simulink model "MySimplifiedTestingModel_20x2810x29"  (R2023a)
settings: Solver=ode1  StartTime=0.0  StopTime=inf  FixedStep=0.001  RelTol=1e-3
PostLoadFcn:
  | , if any(exist('dsrtsu_mdlpostloadfcn', 'file') ~= 0), dsrtsu_mdlpostloadfcn('Execute', bdroot); end,
InitFcn:
  | , if any(exist('rtifpga_mdlclblib', 'file') ~= 0), rtifpga_mdlclblib('Init', bdroot); end,
undefined symbols (not defined in the file or in its folder): START, STOP
libraries: rti1202serlib x11, simulink x6
(part 2 of 3)

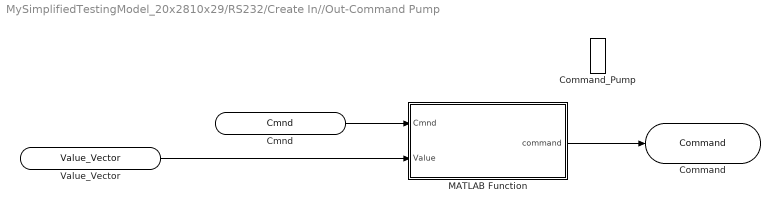
== system MySimplifiedTestingModel_20x2810x29/RS232/Create In//Out-Command Pump ==
  Command_Pump : TriggerPort  TriggerType=function-call  IsSimulinkFunction=on  FunctionName=Command_Pump  VariantControl=(inherit)
  MATLAB Function : MATLAB Function  TreatAsAtomicUnit=on
  Cmnd : ArgIn  ArgumentName=Cmnd
  Value_Vector : ArgIn  Port=2  ArgumentName=Value_Vector
  Command : ArgOut  OutDataTypeStr=uint8  PortDimensions=[1,13]  ArgumentName=Command
  wires:
  Value_Vector/1 -> MATLAB Function/2(Value)
  Cmnd/1 -> MATLAB Function/1(Cmnd)
  MATLAB Function/1(command) -> Command/1

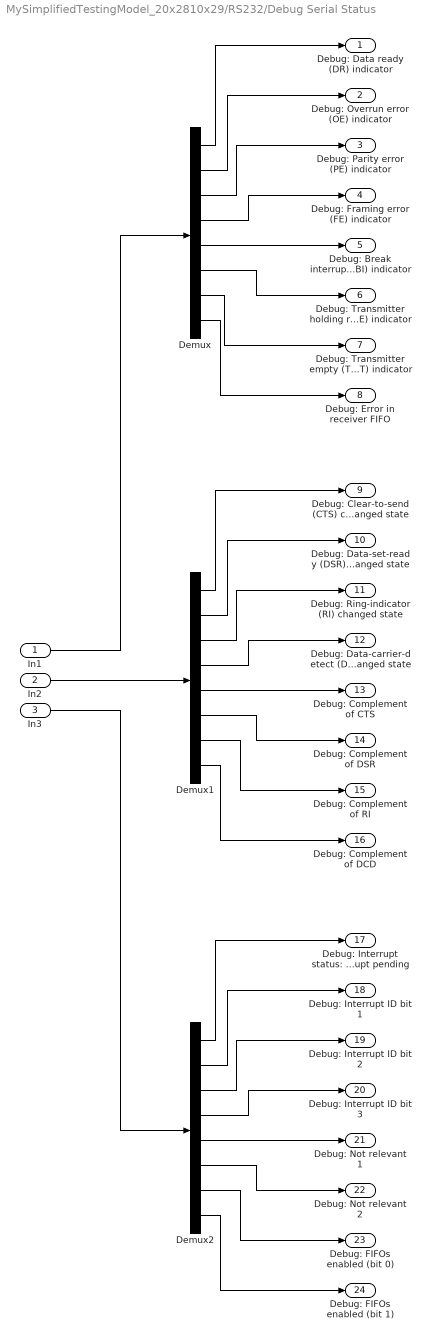
== system MySimplifiedTestingModel_20x2810x29/RS232/Debug Serial Status ==
  In1 : Inport
  In2 : Inport  Port=2
  In3 : Inport  Port=3
  Demux : Demux  Outputs=8
  Demux1 : Demux  Outputs=8
  Demux2 : Demux  Outputs=8
  Debug: Data ready (DR) indicator : Outport
  Debug: Overrun error (OE) indicator : Outport  Port=2
  Debug: Parity error (PE) indicator : Outport  Port=3
  Debug: Framing error (FE) indicator : Outport  Port=4
  Debug: Break interrupt (BI) indicator : Outport  Port=5
  Debug: Transmitter holding register empty (THRE) indicator : Outport  Port=6
  Debug: Transmitter empty (TEMT) indicator : Outport  Port=7
  Debug: Error in receiver FIFO : Outport  Port=8
  Debug: Clear-to-send (CTS) changed state : Outport  Port=9
  Debug: Data-set-ready (DSR) changed state : Outport  Port=10
  Debug: Ring-indicator (RI) changed state : Outport  Port=11
  Debug: Data-carrier-detect (DCD) changed state : Outport  Port=12
  Debug: Complement of CTS : Outport  Port=13
  Debug: Complement of DSR : Outport  Port=14
  Debug: Complement of RI : Outport  Port=15
  Debug: Complement of DCD : Outport  Port=16
  Debug: Interrupt status: 0 if interrupt pending : Outport  Port=17
  Debug: Interrupt ID bit 1 : Outport  Port=18
  Debug: Interrupt ID bit 2 : Outport  Port=19
  Debug: Interrupt ID bit 3 : Outport  Port=20
  Debug: Not relevant 1 : Outport  Port=21
  Debug: Not relevant 2 : Outport  Port=22
  Debug: FIFOs enabled (bit 0) : Outport  Port=23
  Debug: FIFOs enabled (bit 1) : Outport  Port=24
  wires:
  Demux/3 -> Debug: Parity error (PE) indicator/1
  Demux2/4 -> Debug: Interrupt ID bit 3/1
  Demux1/8 -> Debug: Complement of DCD/1
  Demux2/5 -> Debug: Not relevant 1/1
  Demux2/2 -> Debug: Interrupt ID bit 1/1
  Demux/1 -> Debug: Data ready (DR) indicator/1
  In2/1 -> Demux1/1
  Demux1/2 -> Debug: Data-set-ready (DSR) changed state/1
  In1/1 -> Demux/1
  Demux2/7 -> Debug: FIFOs enabled (bit 0)/1
  Demux2/1 -> Debug: Interrupt status: 0 if interrupt pending/1
  Demux2/6 -> Debug: Not relevant 2/1
  Demux2/3 -> Debug: Interrupt ID bit 2/1
  Demux1/7 -> Debug: Complement of RI/1
  Demux1/1 -> Debug: Clear-to-send (CTS) changed state/1
  Demux1/6 -> Debug: Complement of DSR/1
  Demux1/4 -> Debug: Data-carrier-detect (DCD) changed state/1
  Demux1/5 -> Debug: Complement of CTS/1
  Demux1/3 -> Debug: Ring-indicator (RI) changed state/1
  Demux/2 -> Debug: Overrun error (OE) indicator/1
  Demux2/8 -> Debug: FIFOs enabled (bit 1)/1
  Demux/6 -> Debug: Transmitter holding register empty (THRE) indicator/1
  Demux/5 -> Debug: Break interrupt (BI) indicator/1
  Demux/4 -> Debug: Framing error (FE) indicator/1
  Demux/8 -> Debug: Error in receiver FIFO/1
  Demux/7 -> Debug: Transmitter empty (TEMT) indicator/1
  In3/1 -> Demux2/1

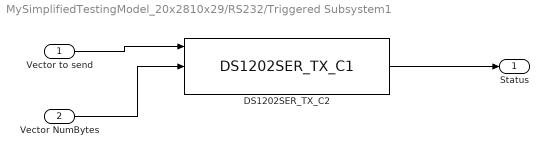
== system MySimplifiedTestingModel_20x2810x29/RS232/Triggered Subsystem1 ==
  Vector to send : Inport
  Vector NumBytes : Inport  Port=2
  DS1202SER_TX_C2 : rti1202serlib/DS1202SER_TX_C1  Reserved1=[]  Reserved2=[]  Reserved3=[]  Reserved4=[]  DSProperties=struct('RTI',struct('IOBoardType',{{'DS1202','SER'}},'SlaveProcessor','NONE','Version',uint32(1),'BlockType',struct('isSLSource',uint8(1),'isSLSink',uint8(1),'isHWSource',uint8(1),'isHWSink',uint8(0),'isSetup',uint8(0),'isInline',uint8(1),'isNonInline',uint8(0),'isInterrupt',uint8(0),'isChannelwise',uint8(1)),'UnitType','GENSER','Identifier','TRANSMIT','DialogType','ML','BlockSet','NONE'))  RTIBlockInterface=struct('BlockName',struct('Token',{{'DS1202SER_TX_C'}},'BlockParam',{{'ChannelNo'}}),'InputPortsWidth',int32([13 1]),'InputPortsActive',[1 1],'InputPortsDataType',{{'SS_UINT8','SS_UINT32'}},'InputPortsName',{{'TXBytes','NumBytes'}},'OutputPortsWidth',int32([1 1]),'OutputPortsActive',[0 1],'OutputPortsDataType',{{'SS_UINT32','SS_INT32'}},'OutputPortsName',{{'NumTXBytes','Status'}},'BlockDisplay',{{['Serial Transmit'],'center'}},'IconTransparency','on','ParameterTunableNames',{{'BytesRefNumOf'}},'InitLevel',2,'DialogFcn','guigensertransmit','MaskDescription',['To write data to the UART SW FIFO.'])  RTIBlockParameters=struct('BoardNo',{{1,'ON',[1 1]}},'ChannelNo',{{2,'ON',[1 2]}},'ChannelNumOf',{{2,'OFF',[]}},'TransmitFifoOverrunMode',{{1,'OFF',[]}},'ParamTunableMode',{{1,'OFF',[]}},'BytesRefNumOfT',{{'1','OFF',[1 inf]}},'BytesRefNumOfNT',{{'1','OFF',[1 inf]}},'BytesRefNumOfMax',{{'13','OFF',[1 inf]}},'BytesRefNumOfMode',{{0,'OFF',[]}},'BytesActNumOfMode',{{0,'OFF',[]}},'TransmissionStatusMode',{{1,'OFF',[]}},'FifoSizeDefault',{{64,'OFF',[]}},'TLCFileName',{{'rtigensertransmit','OFF',[]}})  RTISFcnParameters=struct('BoardNo','double','ChannelNo','double','ChannelNumOf','double','TransmitFifoOverrunMode','double','ParamTunableMode','double','BytesRefNumOfT','double','BytesRefNumOfNT','double','BytesRefNumOfMax','double','BytesRefNumOfMode','double','BytesActNumOfMode','double','TransmissionStatusMode','double','TLCFileName','char')  RTIBlockParaDefault=struct('BoardNo',1,'ChannelNo',1,'ChannelNumOf',2,'TransmitFifoOverrunMode',1,'ParamTunableMode',1,'BytesRefNumOfT',1,'BytesRefNumOfNT',1,'BytesRefNumOfMax',1,'BytesRefNumOfMode',0,'BytesActNumOfMode',1,'TransmissionStatusMode',1,'FifoSizeDefault',64,'TLCFileName','rtigensertransmit')
  Status : Outport
  wires:
  DS1202SER_TX_C2/1 -> Status/1
  Vector NumBytes/1 -> DS1202SER_TX_C2/2
  Vector to send/1 -> DS1202SER_TX_C2/1

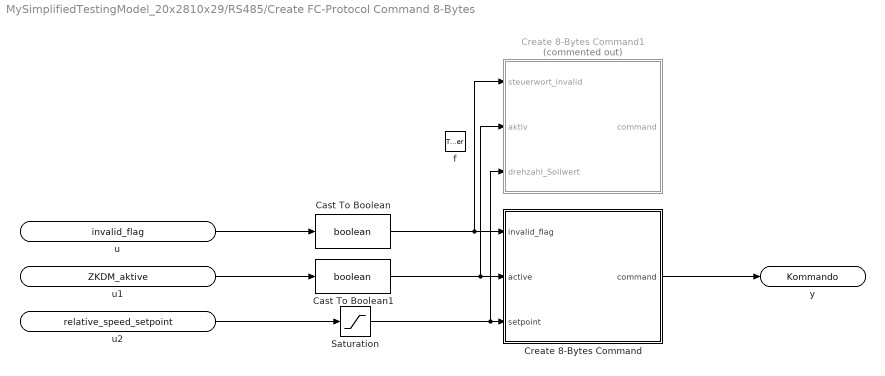
== system MySimplifiedTestingModel_20x2810x29/RS485/Create FC-Protocol Command 8-Bytes ==
  f : TriggerPort  TriggerType=function-call  IsSimulinkFunction=on  FunctionName=FC_Command_8Bytes  VariantControl=(inherit)
  Cast To Boolean : DataTypeConversion  OutDataTypeStr=boolean  SaturateOnIntegerOverflow=off  RndMeth=Floor
  Cast To Boolean1 : DataTypeConversion  OutDataTypeStr=boolean  SaturateOnIntegerOverflow=off  RndMeth=Floor
  Create 8-Bytes Command : MATLAB Function  TreatAsAtomicUnit=on
  Create 8-Bytes Command1 : MATLAB Function  Commented=on  TreatAsAtomicUnit=on
  Saturation : Saturate  UpperLimit=100  LowerLimit=0
  u : ArgIn  DisableCoverage=on  ArgumentName=invalid_flag
  u1 : ArgIn  DisableCoverage=on  Port=2  ArgumentName=ZKDM_aktive
  u2 : ArgIn  DisableCoverage=on  Port=3  ArgumentName=relative_speed_setpoint
  y : ArgOut  DisableCoverage=on  OutDataTypeStr=uint8  PortDimensions=[1, 63]  ArgumentName=Kommando
  wires:
  Saturation/1 -> Create 8-Bytes Command/3(setpoint), Create 8-Bytes Command1/3(drehzahl_Sollwert)
  Cast To Boolean1/1 -> Create 8-Bytes Command/2(active), Create 8-Bytes Command1/2(aktiv)
  Cast To Boolean/1 -> Create 8-Bytes Command/1(invalid_flag), Create 8-Bytes Command1/1(steuerwort_invalid)
  u2/1 -> Saturation/1
  u1/1 -> Cast To Boolean1/1
  u/1 -> Cast To Boolean/1
  Create 8-Bytes Command/1(command) -> y/1

== system MySimplifiedTestingModel_20x2810x29/RS485/Konfiguration für kommunikation ZKDM ==
  Trigger : TriggerPort  VariantControl=(inherit)
  System Outputs : Subsystem  mask(System Outputs){ShowInLibBrowser=0}
      mask prompts: ShowInLibBrowser "Simulink:masks:CustCodeMaskParam1_MP"
      settings: CopyFcn=cccopyfcn(gcb)  OpenFcn=ccopenfcn('System Outputs Function')
      mask Help: eval('feval(''rtwprivate'',''rtwhelpview'',''rtw_sys_outputs_block'')');
      mask DialogControl ShowInLibBrowser Prompt: Mask Parameter 1:
      mask Display: disp('System\nOutputs');

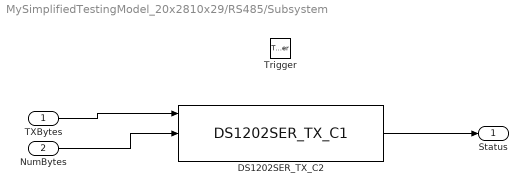
== system MySimplifiedTestingModel_20x2810x29/RS485/Subsystem ==
  TXBytes : Inport
  NumBytes : Inport  Port=2
  Trigger : TriggerPort  VariantControl=(inherit)  PortDimensions=1
  DS1202SER_TX_C2 : rti1202serlib/DS1202SER_TX_C1  Reserved1=[]  Reserved2=[]  Reserved3=[]  Reserved4=[]  DSProperties=struct('RTI',struct('IOBoardType',{{'DS1202','SER'}},'SlaveProcessor','NONE','Version',uint32(1),'BlockType',struct('isSLSource',uint8(1),'isSLSink',uint8(1),'isHWSource',uint8(1),'isHWSink',uint8(0),'isSetup',uint8(0),'isInline',uint8(1),'isNonInline',uint8(0),'isInterrupt',uint8(0),'isChannelwise',uint8(1)),'UnitType','GENSER','Identifier','TRANSMIT','DialogType','ML','BlockSet','NONE'))  RTIBlockInterface=struct('BlockName',struct('Token',{{'DS1202SER_TX_C'}},'BlockParam',{{'ChannelNo'}}),'InputPortsWidth',int32([63 1]),'InputPortsActive',[1 1],'InputPortsDataType',{{'SS_UINT8','SS_UINT32'}},'InputPortsName',{{'TXBytes','NumBytes'}},'OutputPortsWidth',int32([1 1]),'OutputPortsActive',[0 1],'OutputPortsDataType',{{'SS_UINT32','SS_INT32'}},'OutputPortsName',{{'NumTXBytes','Status'}},'BlockDisplay',{{['Serial Transmit'],'center'}},'IconTransparency','on','ParameterTunableNames',{{'BytesRefNumOf'}},'InitLevel',2,'DialogFcn','guigensertransmit','MaskDescription',['To write data to the UART SW FIFO.'])  RTIBlockParameters=struct('BoardNo',{{1,'ON',[1 1]}},'ChannelNo',{{2,'ON',[1 2]}},'ChannelNumOf',{{2,'OFF',[]}},'TransmitFifoOverrunMode',{{1,'OFF',[]}},'ParamTunableMode',{{1,'OFF',[]}},'BytesRefNumOfT',{{'1','OFF',[1 inf]}},'BytesRefNumOfNT',{{'1','OFF',[1 inf]}},'BytesRefNumOfMax',{{'63','OFF',[1 inf]}},'BytesRefNumOfMode',{{0,'OFF',[]}},'BytesActNumOfMode',{{0,'OFF',[]}},'TransmissionStatusMode',{{1,'OFF',[]}},'FifoSizeDefault',{{64,'OFF',[]}},'TLCFileName',{{'rtigensertransmit','OFF',[]}})  RTISFcnParameters=struct('BoardNo','double','ChannelNo','double','ChannelNumOf','double','TransmitFifoOverrunMode','double','ParamTunableMode','double','BytesRefNumOfT','double','BytesRefNumOfNT','double','BytesRefNumOfMax','double','BytesRefNumOfMode','double','BytesActNumOfMode','double','TransmissionStatusMode','double','TLCFileName','char')  RTIBlockParaDefault=struct('BoardNo',1,'ChannelNo',1,'ChannelNumOf',2,'TransmitFifoOverrunMode',1,'ParamTunableMode',1,'BytesRefNumOfT',1,'BytesRefNumOfNT',1,'BytesRefNumOfMax',1,'BytesRefNumOfMode',0,'BytesActNumOfMode',1,'TransmissionStatusMode',1,'FifoSizeDefault',64,'TLCFileName','rtigensertransmit')
  Status : Outport
  wires:
  TXBytes/1 -> DS1202SER_TX_C2/1
  DS1202SER_TX_C2/1 -> Status/1
  NumBytes/1 -> DS1202SER_TX_C2/2

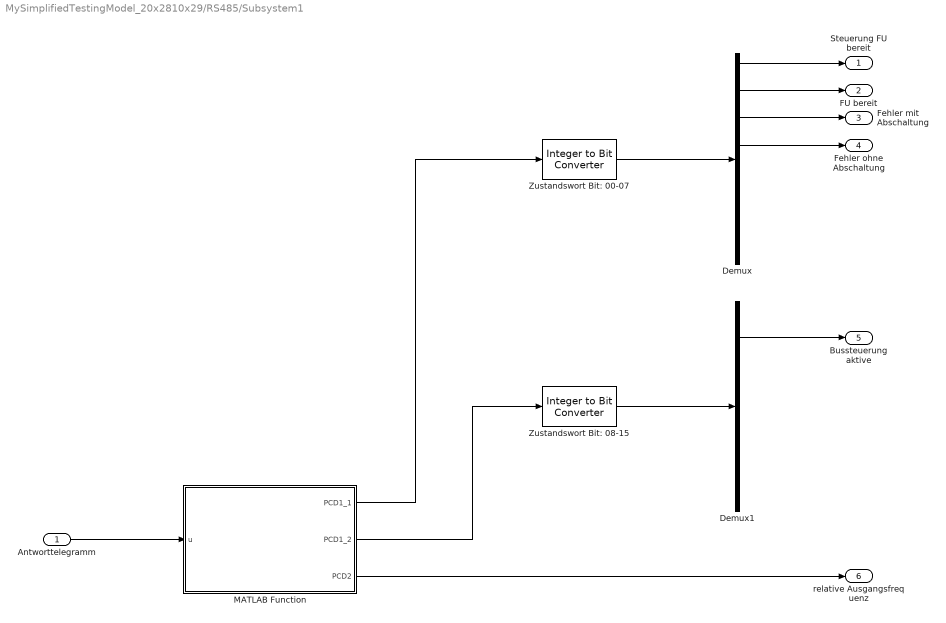
== system MySimplifiedTestingModel_20x2810x29/RS485/Subsystem1 ==
  Antworttelegramm : Inport
  Demux : Demux  Outputs=8
  Demux1 : Demux  Outputs=8
  MATLAB Function : MATLAB Function  TreatAsAtomicUnit=on
  Zustandswort Bit: 00-07 : simulink/Logic and Bit Operations/Integer to Bit Converter  nbits=8  signedInputValues=Unsigned  bitOrder=MSB first  outDtype=boolean
  Zustandswort Bit: 08-15 : simulink/Logic and Bit Operations/Integer to Bit Converter  nbits=8  signedInputValues=Unsigned  bitOrder=MSB first  outDtype=boolean
  Steuerung FU bereit : Outport
  FU bereit : Outport  Port=2
  Fehler mit Abschaltung : Outport  Port=3
  Fehler ohne Abschaltung : Outport  Port=4
  Bussteuerung aktive : Outport  Port=5
  relative Ausgangsfrequenz : Outport  Port=6
  wires:
  MATLAB Function/3(PCD2) -> relative Ausgangsfrequenz/1
  MATLAB Function/2(PCD1_2) -> Zustandswort Bit: 08-15/1
  MATLAB Function/1(PCD1_1) -> Zustandswort Bit: 00-07/1
  Demux1/2 -> Bussteuerung aktive/1
  Zustandswort Bit: 08-15/1 -> Demux1/1
  Zustandswort Bit: 00-07/1 -> Demux/1
  Demux/4 -> Fehler ohne Abschaltung/1
  Demux/3 -> Fehler mit Abschaltung/1
  Demux/2 -> FU bereit/1
  Demux/1 -> Steuerung FU bereit/1
  Antworttelegramm/1 -> MATLAB Function/1(u)

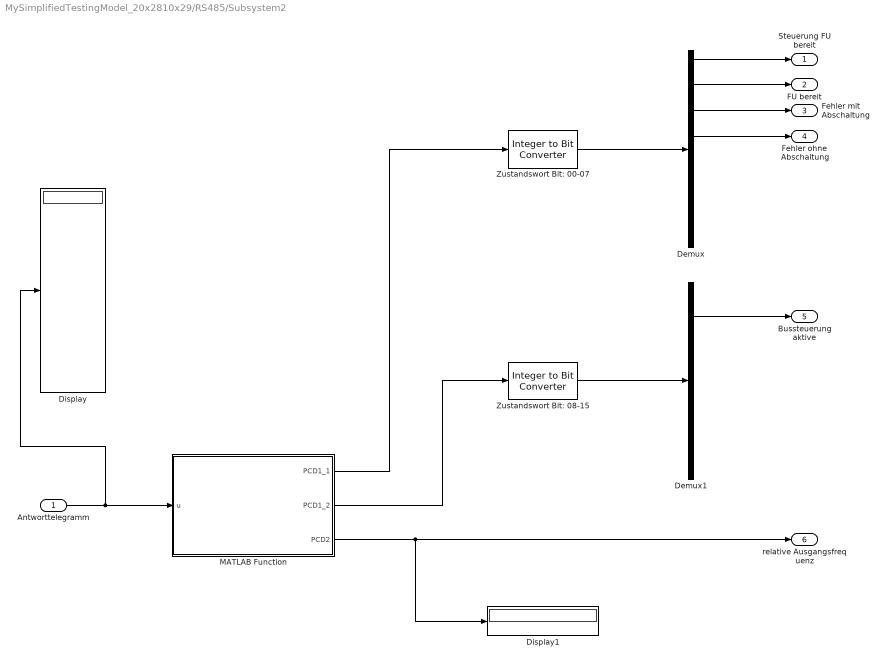
== system MySimplifiedTestingModel_20x2810x29/RS485/Subsystem2 ==
  Antworttelegramm : Inport
  Demux : Demux  Outputs=8
  Demux1 : Demux  Outputs=8
  Display : Display
      settings: Decimation=8
  Display1 : Display
  MATLAB Function : MATLAB Function  TreatAsAtomicUnit=on
  Zustandswort Bit: 00-07 : simulink/Logic and Bit Operations/Integer to Bit Converter  nbits=8  signedInputValues=Unsigned  bitOrder=MSB first  outDtype=boolean
  Zustandswort Bit: 08-15 : simulink/Logic and Bit Operations/Integer to Bit Converter  nbits=8  signedInputValues=Unsigned  bitOrder=MSB first  outDtype=boolean
  Steuerung FU bereit : Outport
  FU bereit : Outport  Port=2
  Fehler mit Abschaltung : Outport  Port=3
  Fehler ohne Abschaltung : Outport  Port=4
  Bussteuerung aktive : Outport  Port=5
  relative Ausgangsfrequenz : Outport  Port=6
  wires:
  MATLAB Function/3(PCD2) -> Display1/1, relative Ausgangsfrequenz/1
  MATLAB Function/2(PCD1_2) -> Zustandswort Bit: 08-15/1
  MATLAB Function/1(PCD1_1) -> Zustandswort Bit: 00-07/1
  Demux1/2 -> Bussteuerung aktive/1
  Zustandswort Bit: 08-15/1 -> Demux1/1
  Zustandswort Bit: 00-07/1 -> Demux/1
  Demux/4 -> Fehler ohne Abschaltung/1
  Demux/3 -> Fehler mit Abschaltung/1
  Demux/2 -> FU bereit/1
  Demux/1 -> Steuerung FU bereit/1
  Antworttelegramm/1 -> Display/1, MATLAB Function/1(u)

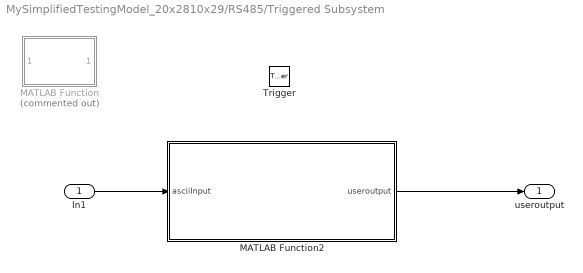
== system MySimplifiedTestingModel_20x2810x29/RS485/Triggered Subsystem ==
  In1 : Inport
  Trigger : TriggerPort  VariantControl=(inherit)
  MATLAB Function : MATLAB Function  Commented=on  TreatAsAtomicUnit=on
  MATLAB Function2 : MATLAB Function  TreatAsAtomicUnit=on
  useroutput : Outport
  wires:
  In1/1 -> MATLAB Function2/1(asciiInput)
  MATLAB Function2/1(useroutput) -> useroutput/1

== system MySimplifiedTestingModel_20x2810x29/RS485/Triggered Subsystem1 ==
  u : Inport
  Trigger : TriggerPort  VariantControl=(inherit)
  MATLAB Function : MATLAB Function  TreatAsAtomicUnit=on
  y : Outport
  wires:
  u/1 -> MATLAB Function/1(command)
  MATLAB Function/1(userFriendlyOutput) -> y/1

== system MySimplifiedTestingModel_20x2810x29/RTI Data/RTI Data Store ==
  RTI Data Store : Subsystem  mask(RTI_DATA_STORE){}
      mask help:
      | RTI Data Store Block. This block is used by RTI to store internal model dependent data. Deleting this block will result in data loss.
      |
      | NEVER DELETE, COPY, OR MODIFY THIS BLOCK!
      mask Help:
      | RTI Data Store Block. This block is used by RTI to store internal model dependent data. Deleting this block will result in data loss.
      | 
      | NEVER DELETE, COPY, OR MODIFY THIS BLOCK!
      mask Display: text(0.5, 0.5, ' ', 'HorizontalAlignment', 'center');

== system MySimplifiedTestingModel_20x2810x29/RS485/Konfiguration für kommunikation ZKDM/System Outputs ==

== system MySimplifiedTestingModel_20x2810x29/RTI Data/RTI Data Store/RTI Data Store ==
  RTI Data Store : Subsystem  mask(RTI_DATA_STORE){}
      mask help:
      | RTI Data Store Block. This block is used by RTI to store internal model dependent data. Deleting this block will result in data loss.
      |
      | NEVER DELETE, COPY, OR MODIFY THIS BLOCK!
      mask Help:
      | RTI Data Store Block. This block is used by RTI to store internal model dependent data. Deleting this block will result in data loss.
      | 
      | NEVER DELETE, COPY, OR MODIFY THIS BLOCK!
      mask Display: text(0.5, 0.5, ' ', 'HorizontalAlignment', 'center');

== system MySimplifiedTestingModel_20x2810x29/RTI Data/RTI Data Store/RTI Data Store/RTI Data Store ==
  RTI Data Store : Subsystem  mask(RTI_DATA_STORE){}
      mask help:
      | RTI Data Store Block. This block is used by RTI to store internal model dependent data. Deleting this block will result in data loss.
      |
      | NEVER DELETE, COPY, OR MODIFY THIS BLOCK!
      mask Help:
      | RTI Data Store Block. This block is used by RTI to store internal model dependent data. Deleting this block will result in data loss.
      | 
      | NEVER DELETE, COPY, OR MODIFY THIS BLOCK!
      mask Display: text(0.5, 0.5, ' ', 'HorizontalAlignment', 'center');

== system MySimplifiedTestingModel_20x2810x29/RTI Data/RTI Data Store/RTI Data Store/RTI Data Store/RTI Data Store ==

== matlab function MySimplifiedTestingModel_20x2810x29/RS485/Subsystem2/MATLAB Function ==
  data: u input; PCD1_1 output; PCD1_2 output; PCD2 output
function [PCD1_1, PCD1_2, PCD2] = fcn(u)
%Steuerwort
PCD1_1 = u(4);
PCD1_2 = u(5);

%berechnet aktuelle Ausgangsfrequenz als relativen Wert in Prozent
PCD2 = (u(6)*256 + u(7)) * (100 / 16384);

== matlab function MySimplifiedTestingModel_20x2810x29/RS485/MATLAB Function3 ==
  data: fu_ctrl_ready input; u output; fu_ready input; fault_trip input; fault_no_trip input; bus_control_active input; freq_rel_percent input; addr input
function u = build_fc_rx_telegram(fu_ctrl_ready, fu_ready, fault_trip, fault_no_trip, bus_control_active, freq_rel_percent, addr)
%#codegen
% Build an 8-byte Danfoss FC "reply" telegram:
%   [STX, LEN, ADDR, STW_HI, STW_LO, OUT_HI, OUT_LO, BCC]
%
% Inputs:
%   fu_ctrl_ready       : logical  % maps to STW bit 0
%   fu_ready            : logical  % maps to STW bit 1
%   fault_trip          : logical  % maps to STW bit 2 (trip = hard fault)
%   fault_no_trip       : logical  % maps to STW bit 3 (warning)
%   bus_control_active  : logical  % maps to STW bit 12
%   freq_rel_percent    : double   % 0..100 (%) — will be clamped & rounded to Q14
%   addr                : uint8    % (optional) on-wire FC address byte; default 253
%
% Output:
%   u (1x8 uint8) = FC reply frame you can feed into your parser
%
% Notes:
% - Mapping follows the demo you showed:
%     bit0 = fu_ctrl_ready
%     bit1 = fu_ready
%     bit2 = fault_trip
%     bit3 = fault_no_trip
%     bit12 = bus_control_active
% - OUT is Q14: 0..16384 ↔ 0..100%

    if nargin < 7
        addr = uint8(253);   % default FC on-wire address (e.g., node 125)
    else
        addr = uint8(addr);
    end

    % helper: convert MSB index k (15..0) to bitset() position (1..16)
    msbpos = @(k) 16 - k;
    
    sw = uint16(0);
    if fu_ctrl_ready,      sw = bitset(sw, msbpos(0),  true); end   % bit0
    if fu_ready,           sw = bitset(sw, msbpos(1),  true); end   % bit1
    if fault_trip,         sw = bitset(sw, msbpos(2),  true); end   % bit2
    if fault_no_trip,      sw = bitset(sw, msbpos(3),  true); end   % bit3
    if bus_control_active, sw = bitset(sw, msbpos(9),  true); end   % bit9

    STW_HI = uint8(bitshift(sw, -8));
    STW_LO = uint8(bitand(sw, 255));

    % ---------- OUT (Q14) from percent ----------
    if ~isfinite(freq_rel_percent), freq_rel_percent = 0; end
    freq_rel_percent = max(0, min(100, freq_rel_percent));
    q14 = uint16(round(freq_rel_percent * (16384/100)));
    OUT_HI = uint8(bitshift(q14, -8));
    OUT_LO = uint8(bitand(q14, 255));

    % ---------- assemble frame ----------
    STX = uint8(2);
    LEN = uint8(6);   % addr + 4 data bytes + BCC

    u = zeros(1,8,'uint8');
    u(1) = STX;
    u(2) = LEN;
    u(3) = addr;
    u(4) = STW_HI;
    u(5) = STW_LO;
    u(6) = OUT_HI;
    u(7) = OUT_LO;

    % ---------- BCC (XOR of bytes 1..7) ----------
    bcc = uint8(0);
    for k = 1:7
        bcc = bitxor(bcc, u(k));
    end
    u(8) = bcc;
end

== matlab function MySimplifiedTestingModel_20x2810x29/RS232/Create In//Out-Command Pump/MATLAB Function ==
  data: command output; Cmnd input; Value input

function command = fcn(Cmnd, Value)
    % Initialize the command array with zeros
    command = zeros(1, 13, 'uint8'); % Pre-allocate for fixed-length command

    % Create the RS232 command based on the 'Cmnd' input
    switch Cmnd
        case 0
            % "START" command
            command(1:5) = uint8('START');
            command(6) = uint8(13); % Carriage return
            command(7) = uint8(10); % Line feed

        case 1
            % "STOP" command
            command(1:4) = uint8('STOP');
            command(5) = uint8(13); % Carriage return
            command(6) = uint8(10); % Line feed

        case 2
            % "OUT_SP_1" command - to set the setpoint
            command(1:8) = uint8('OUT_SP_1');

            % Convert Value to int32 to ensure it's an integer type
                       
            % Ensure Value is int32 
                      
            % Ensure Value is int32 
            value_int = Value;
            
            % Preallocate an array for three digits
            digits = zeros(1, 3, 'uint8'); 
            
            % Fill the digits directly, ensuring leading zeros are accounted for
            digits(1) = uint8(floor(mod(value_int, 1000) / 100)); % Hundreds place
            digits(2) = uint8(floor(mod(value_int, 100) / 10));   % Tens place
            digits(3) = uint8(mod(value_int, 10));                 % Ones place
            
            % Convert digits to character codes by adding ASCII '0'
            command(9:11) = digits + uint8('0'); % Assign ASCII values for the digits
            
            % Alternatively, you can individually convert to character codes
            % command(9) = uint8(digits(1) + '0'); % Hundreds
            % command(10) = uint8(digits(2) + '0'); % Tens
            % command(11) = uint8(digits(3) + '0'); % Ones

            % Place carriage return and line feed
            command(12) = uint8(13); % Carriage return
            command(13) = uint8(10); % Line feed

        case 3
            % "IN_PV_1" command - to read the actual value
            command(1:7) = uint8('IN_PV_1');
            command(8) = uint8(13); % Carriage return
            command(9) = uint8(10); % Line feed

        case 4
            % "STATUS" command - to ask for the status
            command(1:6) = uint8('STATUS');
            command(7) = uint8(13); % Carriage return
            command(8) = uint8(10); % Line feed

        otherwise
            error('Invalid command: Cmnd must be an integer between 0 and 4.');
    end
end

== matlab function MySimplifiedTestingModel_20x2810x29/RS485/Create 8-Bytes Command ==
  data: invalid_flag input; active input; command output; setpoint input
% Generates a telegram of the FC protocol for communication with a Danfoss frequency converter,
% telegram type: Process block (PCD) – 4 bytes
%
%##################################################################################
%Danfoss control word according to FC profile
%----------------------------------------------------------------------------------
%| Bit|                        Bit value = 0 |                     Bit value = 1  |
%|----|--------------------------------------|------------------------------------|
%| 00 | selection between the four "3-10 Preset reference [0]...[3]"             |
%| 01 | --""--                                                                   |
%|----|--------------------------------------|------------------------------------|
%| 02 |             DC brake and stop        |             performs ramp          |
%|----|--------------------------------------|------------------------------------|
%| 03 | lets the motor coast                 | starts the motor if conditions are met |
%|----|--------------------------------------|------------------------------------|
%| 04 | motor speed decreases until stop     |                                    |
%|----|--------------------------------------|------------------------------------|
%| 05 | current output frequency is stored   |                                    |
%|----|--------------------------------------|------------------------------------|
%| 06 | stop using ramp time                 | starts the motor if conditions are met |
%|----|--------------------------------------|------------------------------------|
%| 07 | no reset                             | reset                              |
%|----|--------------------------------------|------------------------------------|
%| 08 |                                      | output frequency "3-19 Jog [RPM]"  |
%|----|--------------------------------------|------------------------------------|
%| 09 | ramp 1 active ("3-41" and "3-42")    | ramp 2 active ("3-51" and "3-52")  |
%|----|--------------------------------------|------------------------------------|
%| 10 | control word is ignored              | control word is used               |
%|----|--------------------------------------|------------------------------------|
%| 11 | relay 01 not activated               | relay 01 activated                 |
%|----|--------------------------------------|------------------------------------|
%| 12 | relay 04 not activated               | relay 04 activated                 |
%|----|--------------------------------------|------------------------------------|
%| 13 | parameter set selection "0-10" and "8-55"                                |
%| 14 |                                                                            |
%|----|--------------------------------------|------------------------------------|
%| 15 | no reversal                          | reversal                           |
%----------------------------------------------------------------------------------
%##################################################################################

function command = fcn(invalid_flag, active, setpoint)

if setpoint < 0
        error('setpoint must be non-negative.');
end

command = zeros(1, 64, 'uint8');
startzeichen = uint8(2);    % Start character (STX)
telegrammlaenge = uint8(6); % Specifies telegram length: 6 or 14 data bytes (data bytes + address byte + checksum)
adresse = 0b01111101;       % Address 125 in binary, address of the frequency converter (FU)
                            % Address format 1–126 => Bit 7 = 1; FU address “10” => Bit 0–6
pcd1_1 = 0b00000000;        % Control word (CTW) bits 08 to 15
pcd1_2 = 0b00101110;        % Control word (CTW) bits 00 to 07
bcc = 0;                    % Data control byte, Block Check Character (BCC)

% modify the flag
if (invalid_flag == false)
    pcd1_1 = bitor(pcd1_1, 0b00100000); 
    % If invalid_flag is `false`, the result will change `pcd11` to `0b00100000`, indicating that the control word is now in use.
end

if (active == true)
    pcd1_1 = bitor(pcd1_1, 0b00010000); % Starts the motor; “0”: the frequency converter lets the motor coast
end

%%- `command(4) = pcd1_1;`
  % - Value: This byte is constructed based on the input conditions (`steuerwort_invalid` and `aktiv`).
  % - It starts with `0b00000000` (initial value) and may have bits set:
  %   - Bit 5 is set to 1 if `steuerwort_invalid` is false (valid control word).
  %   - Bit 4 is set to 1 if `aktiv` is true (start command).
  % - As a result, if `aktiv` is true, the value changes:
  %     - From: `0b00100000`
  %     - To:   `0b00110000` (decimal 48), indicating that the motor should start.

% scale the speed setpoint
% Example: convert 50% speed to 16-bit integer
% 50% = (16384 / 100 * 50) = 8192
% 8192 = 0b1000000000000000 (binary)

soll = setpoint * (16384 / 100); 
pcd2 = typecast(int16(soll),'uint8');
pcd2 = flip(pcd2);
%This is a 16-bit integer converted to two bytes that represents the desired speed (drehzahl_Sollwert) scaled to a proper range.
   %- The speed is scaled by multiplying the `drehzahl_Sollwert` by `(16384 / 100)`, allowing for a representation of the speed setting as a 16-bit integer.
   %- This is then converted from an `int16` to `uint8`, giving two bytes: `pcd2(1)` and `pcd2(2)`, with the bytes being flipped to match byte order expectations.

bcc = bitxor(startzeichen, telegrammlaenge);
bcc = bitxor(bcc, adresse);
bcc = bitxor(bcc, pcd1_1);
bcc = bitxor(bcc, pcd1_2);
bcc = bitxor(bcc, pcd2(1));
bcc = bitxor(bcc, pcd2(2));

command(1) = startzeichen;
command(2) = telegrammlaenge;
command(3) = adresse;
command(4) = pcd1_1; %This byte functions as part of the control command to the motor, determining how it should behave.
command(5) = pcd1_2; %This byte also forms part of the control command. It usually contains predefined flags or control commands as per the motor's specification.
command(6:7) = pcd2; %This part of the command specifies the desired speed for the motor. from the user sollwert.
command(8) = bcc;

%example message:

%Address: 118 Motor Activation Flag: True Target Speed: 89% BCC is valid
%2 6 118 48 46 56 246 162

== matlab function MySimplifiedTestingModel_20x2810x29/RS485/MATLAB Function4 ==
  data: fu_ctrl_ready input; u output; fu_ready input; fault_trip input; fault_no_trip input; bus_control_active input; freq_rel_percent input; addr input
function u = build_fc_rx_telegram(fu_ctrl_ready, fu_ready, fault_trip, fault_no_trip, bus_control_active, freq_rel_percent, addr)
%#codegen
% Build an 8-byte Danfoss FC "reply" telegram:
%   [STX, LEN, ADDR, STW_HI, STW_LO, OUT_HI, OUT_LO, BCC]
%
% Inputs:
%   fu_ctrl_ready       : logical  % maps to STW bit 0
%   fu_ready            : logical  % maps to STW bit 1
%   fault_trip          : logical  % maps to STW bit 2 (trip = hard fault)
%   fault_no_trip       : logical  % maps to STW bit 3 (warning)
%   bus_control_active  : logical  % maps to STW bit 12
%   freq_rel_percent    : double   % 0..100 (%) — will be clamped & rounded to Q14
%   addr                : uint8    % (optional) on-wire FC address byte; default 253
%
% Output:
%   u (1x8 uint8) = FC reply frame you can feed into your parser
%
% Notes:
% - Mapping follows the demo you showed:
%     bit0 = fu_ctrl_ready
%     bit1 = fu_ready
%     bit2 = fault_trip
%     bit3 = fault_no_trip
%     bit12 = bus_control_active
% - OUT is Q14: 0..16384 ↔ 0..100%

    if nargin < 7
        addr = uint8(253);   % default FC on-wire address (e.g., node 125)
    else
        addr = uint8(addr);
    end

    % helper: convert MSB index k (15..0) to bitset() position (1..16)
    msbpos = @(k) 16 - k;
    
    sw = uint16(0);
    if fu_ctrl_ready,      sw = bitset(sw, msbpos(0),  true); end   % bit0
    if fu_ready,           sw = bitset(sw, msbpos(1),  true); end   % bit1
    if fault_trip,         sw = bitset(sw, msbpos(2),  true); end   % bit2
    if fault_no_trip,      sw = bitset(sw, msbpos(3),  true); end   % bit3
    if bus_control_active, sw = bitset(sw, msbpos(9),  true); end   % bit9

    STW_HI = uint8(bitshift(sw, -8));
    STW_LO = uint8(bitand(sw, 255));

    % ---------- OUT (Q14) from percent ----------
    if ~isfinite(freq_rel_percent), freq_rel_percent = 0; end
    freq_rel_percent = max(0, min(100, freq_rel_percent));
    q14 = uint16(round(freq_rel_percent * (16384/100)));
    OUT_HI = uint8(bitshift(q14, -8));
    OUT_LO = uint8(bitand(q14, 255));

    % ---------- assemble frame ----------
    STX = uint8(2);
    LEN = uint8(6);   % addr + 4 data bytes + BCC

    u = zeros(1,64,'uint8');
    u(1) = STX;
    u(2) = LEN;
    u(3) = addr;
    u(4) = STW_HI;
    u(5) = STW_LO;
    u(6) = OUT_HI;
    u(7) = OUT_LO;

    % ---------- BCC (XOR of bytes 1..7) ----------
    bcc = uint8(0);
    for k = 1:7
        bcc = bitxor(bcc, u(k));
    end
    u(8) = bcc;
end

== matlab function MySimplifiedTestingModel_20x2810x29/RS485/Triggered Subsystem/MATLAB Function2 ==
  data: asciiInput input; useroutput output

function useroutput = decode_command(asciiInput)
    % Ensure asciiInput is not empty
    if isempty(asciiInput)
        useroutput = "Input is empty. Please provide a valid command string.";
        return;  % Exit function for empty input
    end
    
    % Convert ASCII values to a character string
    commandStr = char(asciiInput);  % Convert the ASCII input to a character string

    % Trim the command string to remove leading or trailing whitespace
    commandStr = strtrim(commandStr);

    % Debugging output (to see the trimmed command string)
    disp(['Command String for Decoding: "' commandStr '"']);  % Use disp instead of fprintf for Simulink

    % Find the position of the first space
    spaceIndices = strfind(commandStr, ' ');
    
    % Check if there are enough parts (at least one space for two parts)
    if numel(spaceIndices) < 1
        useroutput = "Invalid command format: Not enough parts to extract address and command.";
        return;  % Exit function for invalid format
    end

    % The first part is the combined address and command
    addressCommand = commandStr(1:spaceIndices(1)-1);  % Get first part up to the first space

    % Extract the address
    address = extractAddress(addressCommand);

    % Extract the command
    command = extractCommand(addressCommand);
    disp(['Extracted Address: "' address '"']);
    disp(['Extracted Command: "' command '"']);

    % Initialize the set point value
    setPoint = NaN;  % Default to NaN if not provided

    % Check if there's a second part for the set point
    if numel(spaceIndices) > 1
        setPointStr = strtrim(commandStr(spaceIndices(1)+1:end));  % Get everything after the first space
        setPoint = str2double(setPointStr);  % Convert the set point from string to double
    end

    % Construct the output message as a string
    if isnan(setPoint)
        useroutput = "Address: " + address + ", Command: " + command + ", Set Point: Not Provided";
    else
        useroutput = "Address: " + address + ", Command: " + command + ", Set Point: " + string(setPoint);
    end
end

function address = extractAddress(addressCommand)
    % Extract the first four characters for the address
    address = addressCommand(1:5);
end

function command = extractCommand(addressCommand)
    % Extract everything after the first four characters as a command
    command = addressCommand(6:end);
end

== matlab function MySimplifiedTestingModel_20x2810x29/RS485/Create FC-Protocol Command 8-Bytes/Create 8-Bytes Command ==
  data: invalid_flag input; active input; command output; setpoint input
% Generates a telegram of the FC protocol for communication with a Danfoss frequency converter,
% telegram type: Process block (PCD) – 4 bytes
%
%##################################################################################
%Danfoss control word according to FC profile
%----------------------------------------------------------------------------------
%| Bit|                        Bit value = 0 |                     Bit value = 1  |
%|----|--------------------------------------|------------------------------------|
%| 00 | selection between the four "3-10 Preset reference [0]...[3]"             |
%| 01 | --""--                                                                   |
%|----|--------------------------------------|------------------------------------|
%| 02 |             DC brake and stop        |             performs ramp          |
%|----|--------------------------------------|------------------------------------|
%| 03 | lets the motor coast                 | starts the motor if conditions are met |
%|----|--------------------------------------|------------------------------------|
%| 04 | motor speed decreases until stop     |                                    |
%|----|--------------------------------------|------------------------------------|
%| 05 | current output frequency is stored   |                                    |
%|----|--------------------------------------|------------------------------------|
%| 06 | stop using ramp time                 | starts the motor if conditions are met |
%|----|--------------------------------------|------------------------------------|
%| 07 | no reset                             | reset                              |
%|----|--------------------------------------|------------------------------------|
%| 08 |                                      | output frequency "3-19 Jog [RPM]"  |
%|----|--------------------------------------|------------------------------------|
%| 09 | ramp 1 active ("3-41" and "3-42")    | ramp 2 active ("3-51" and "3-52")  |
%|----|--------------------------------------|------------------------------------|
%| 10 | control word is ignored              | control word is used               |
%|----|--------------------------------------|------------------------------------|
%| 11 | relay 01 not activated               | relay 01 activated                 |
%|----|--------------------------------------|------------------------------------|
%| 12 | relay 04 not activated               | relay 04 activated                 |
%|----|--------------------------------------|------------------------------------|
%| 13 | parameter set selection "0-10" and "8-55"                                |
%| 14 |                                                                            |
%|----|--------------------------------------|------------------------------------|
%| 15 | no reversal                          | reversal                           |
%----------------------------------------------------------------------------------
%##################################################################################

function command = fcn(invalid_flag, active, setpoint)

if setpoint < 0
        error('setpoint must be non-negative.');
end

command = zeros(1, 63, 'uint8');
startzeichen = uint8(2);    % Start character (STX)
telegrammlaenge = uint8(6); % Specifies telegram length: 6 or 14 data bytes (data bytes + address byte + checksum)
adresse = 0b01111101;       % Address 125 in binary, address of the frequency converter (FU)
                            % Address format 1–126 => Bit 7 = 1; FU address “10” => Bit 0–6
pcd1_1 = 0b00000000;        % Control word (CTW) bits 08 to 15
pcd1_2 = 0b00101110;        % Control word (CTW) bits 00 to 07
bcc = 0;                    % Data control byte, Block Check Character (BCC)

% modify the flag
if (invalid_flag == false)
    pcd1_1 = bitor(pcd1_1, 0b00100000); 
    % If invalid_flag is `false`, the result will change `pcd11` to `0b00100000`, indicating that the control word is now in use.
end

if (active == true)
    pcd1_1 = bitor(pcd1_1, 0b00010000); % Starts the motor; “0”: the frequency converter lets the motor coast
end

%%- `command(4) = pcd1_1;`
  % - Value: This byte is constructed based on the input conditions (`steuerwort_invalid` and `aktiv`).
  % - It starts with `0b00000000` (initial value) and may have bits set:
  %   - Bit 5 is set to 1 if `steuerwort_invalid` is false (valid control word).
  %   - Bit 4 is set to 1 if `aktiv` is true (start command).
  % - As a result, if `aktiv` is true, the value changes:
  %     - From: `0b00100000`
  %     - To:   `0b00110000` (decimal 48), indicating that the motor should start.

% scale the speed setpoint
% Example: convert 50% speed to 16-bit integer
% 50% = (16384 / 100 * 50) = 8192
% 8192 = 0b1000000000000000 (binary)

soll = setpoint * (16384 / 100); 
pcd2 = typecast(int16(soll),'uint8');
pcd2 = flip(pcd2);
%This is a 16-bit integer converted to two bytes that represents the desired speed (drehzahl_Sollwert) scaled to a proper range.
   %- The speed is scaled by multiplying the `drehzahl_Sollwert` by `(16384 / 100)`, allowing for a representation of the speed setting as a 16-bit integer.
   %- This is then converted from an `int16` to `uint8`, giving two bytes: `pcd2(1)` and `pcd2(2)`, with the bytes being flipped to match byte order expectations.

bcc = bitxor(startzeichen, telegrammlaenge);
bcc = bitxor(bcc, adresse);
bcc = bitxor(bcc, pcd1_1);
bcc = bitxor(bcc, pcd1_2);
bcc = bitxor(bcc, pcd2(1));
bcc = bitxor(bcc, pcd2(2));

command(1) = startzeichen;
command(2) = telegrammlaenge;
command(3) = adresse;
command(4) = pcd1_1; %This byte functions as part of the control command to the motor, determining how it should behave.
command(5) = pcd1_2; %This byte also forms part of the control command. It usually contains predefined flags or control commands as per the motor's specification.
command(6:7) = pcd2; %This part of the command specifies the desired speed for the motor. from the user sollwert.
command(8) = bcc;

%example message:

%Address: 118 Motor Activation Flag: True Target Speed: 89% BCC is valid
%2 6 118 48 46 56 246 162

== stateflow chart MySimplifiedTestingModel_20x2810x29/RS232/Chart ==
  state Modeselection
  state PUMP [group]
    state StartStop
      en: on = true;
      en: prev2= Value_numeric;
      en:
      if Pump_Start_Stop == true
      [Command] = Command_Pump(0,0);
      else
      [Command] = Command_Pump(1,0);
      end
    state Value
      en: prev2 = Value_numeric;
      en: on= true;
      en:
      [Command] = Command_Pump(2, double(Value_numeric));
    state Wait
      en: prev1 = Pump_Start_Stop;
      en: on= false;
    Wait -> StartStop [order 2] : [(Pump_Start_Stop ~= prev1)]
    Value -> Wait : [after(1,sec)]
    StartStop -> Wait : [after(1,sec)]
    Wait -> Value [order 1] : [(Pump_Start_Stop == true && Value_numeric ~= prev2) ]
  (default) -> Modeselection
  Modeselection -> StartStop : [mode == 0]
  data: Pump_Start_Stop input; Value_numeric input; mode input; Command output uint8 size=[1,13]; prev1 local; prev2 local; on output

== matlab function MySimplifiedTestingModel_20x2810x29/RS485/Triggered Subsystem/MATLAB Function ==
  data: asciiInput input; useroutput output

function useroutput = decode_command(asciiInput)
    % Ensure asciiInput is not empty
    if isempty(asciiInput)
        useroutput = "Input is empty. Please provide a valid command string.";
        return;  % Exit function for empty input
    end
    
    % Convert ASCII values to a character string
    commandStr = char(asciiInput);  % Convert the ASCII input to a character string

    % Trim the command string to remove leading or trailing whitespace
    commandStr = strtrim(commandStr);

    % Debugging output (to see the trimmed command string)
    disp(['Command String for Decoding: "' commandStr '"']);  % Use disp instead of fprintf for Simulink

    % Find the position of the first space
    spaceIndices = strfind(commandStr, ' ');
    
    % Check if there are enough parts (at least one space for two parts)
    if numel(spaceIndices) < 1
        useroutput = "Invalid command format: Not enough parts to extract address and command.";
        return;  % Exit function for invalid format
    end

    % The first part is the combined address and command
    addressCommand = commandStr(1:spaceIndices(1)-1);  % Get first part up to the first space

    % Extract the address
    address = extractAddress(addressCommand);

    % Extract the command
    command = extractCommand(addressCommand);
    disp(['Extracted Address: "' address '"']);
    disp(['Extracted Command: "' command '"']);

    % Initialize the set point value
    setPoint = NaN;  % Default to NaN if not provided

    % Check if there's a second part for the set point
    if numel(spaceIndices) > 1
        setPointStr = strtrim(commandStr(spaceIndices(1)+1:end));  % Get everything after the first space
        setPoint = str2double(setPointStr);  % Convert the set point from string to double
    end

    % Construct the output message as a string
    if isnan(setPoint)
        useroutput = "Address: " + address + ", Command: " + command + ", Set Point: Not Provided";
    else
        useroutput = "Address: " + address + ", Command: " + command + ", Set Point: " + string(setPoint);
    end
end

function address = extractAddress(addressCommand)
    % Extract the first four characters for the address
    address = addressCommand(1:5);
end

function command = extractCommand(addressCommand)
    % Extract everything after the first four characters as a command
    command = addressCommand(6:end);
end

== matlab function MySimplifiedTestingModel_20x2810x29/RS485/Triggered Subsystem1/MATLAB Function ==
  data: command input; userFriendlyOutput output

function userFriendlyOutput = interpretCommand(command)
    % Function to interpret generated RS485 command and convert to user-friendly format
    % Input: command is a vector (1x8) with byte values in uint8
    % Output: userFriendlyOutput is a string describing the command in understandable terms
    
    userFriendlyOutput = ''; % Initialize output

    % Ensure the command length is correct
    if length(command) < 8
        userFriendlyOutput = 'Command is not complete.';
        return;
    end

    % Extracting each byte from the command
    stx = command(1); % Start of Text (should be 2)
    lengthOfTelegram = command(2); % Length byte
    address = command(3); % Address byte
    controlWord = command(4); % Control word byte
    additionalByte = command(5); % Unused or additional byte
    speedLSB = command(6); % Least Significant Byte of speed
    speedMSB = command(7); % Most Significant Byte of speed
    bcc = command(8); % Block Check Character (BCC)
    
    
    % Verify STX
    if stx ~= 2
        userFriendlyOutput = strcat(userFriendlyOutput, sprintf('Warning: STX is not correct. Expected: 2. Found: %d\n', stx));
    end

    % Verify Length
    if lengthOfTelegram ~= 6
        userFriendlyOutput = strcat(userFriendlyOutput, sprintf('Warning: Length of telegram is not correct. Expected: 6. Found: %d\n', lengthOfTelegram));
    end

    % Address Interpretation
    userFriendlyOutput = strcat(userFriendlyOutput, sprintf('Address: %d\n', address));

    % Control Word Interpretation
    switch controlWord
        case 32
            userFriendlyOutput = strcat(userFriendlyOutput, 'Motor Activation Flag: False\n');
        case 48
            userFriendlyOutput = strcat(userFriendlyOutput, 'Motor Activation Flag: True\n');
        otherwise
            userFriendlyOutput = strcat(userFriendlyOutput, 'Control word does not determine motor activation: STATUS Feedback\n');
    end

    % Speed Calculation
    speed = typecast(uint8([speedMSB, speedLSB]), 'int16'); % Combine bytes to form the speed value
    drehzahl_Sollwert = round(double(speed) * 100 / 16384); % Convert the raw speed back to percentage
    userFriendlyOutput = strcat(userFriendlyOutput, sprintf('Target Speed: %d%%\n', drehzahl_Sollwert));

    % Block Check Character Calculation
    calculatedBCC = bitxor(stx, lengthOfTelegram);   % Start with STX and Length
    calculatedBCC = bitxor(calculatedBCC, address);  % XOR with Address
    calculatedBCC = bitxor(calculatedBCC, controlWord); % XOR with Control Word
    calculatedBCC = bitxor(calculatedBCC, additionalByte); % XOR with additional byte
    calculatedBCC = bitxor(calculatedBCC, speedLSB); % XOR with LSB of speed
    calculatedBCC = bitxor(calculatedBCC, speedMSB); % XOR with MSB of speed

    % Verify BCC
    if bcc ~= calculatedBCC
        userFriendlyOutput = strcat(userFriendlyOutput, sprintf('Warning: BCC does not match. Expected: %d, Found: %d\n', calculatedBCC, bcc));
    else
        userFriendlyOutput = strcat(userFriendlyOutput, 'BCC is valid\n');
    end
end
